simulink model "ModeloBloque"  (R2013a)
settings: Solver=ode45  StartTime=0.0  StopTime=300  RelTol=1e-3
settings Model: Creator=Cristhian Ivan  LastModifiedBy=Cristhian Ivan

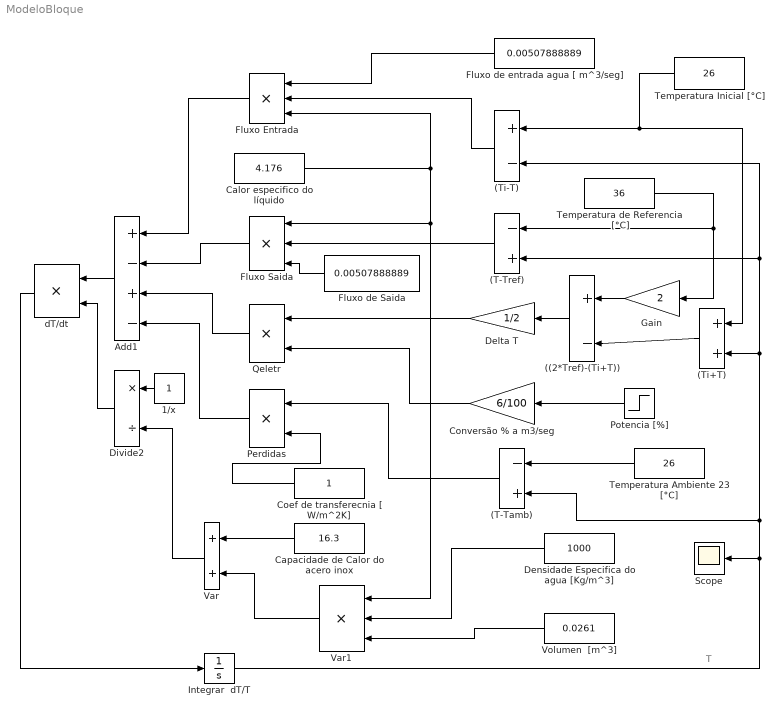
== system ModeloBloque ==
  note: T
  ((2*Tref)-(Ti+T)) : Sum  Inputs=+-
  (T-Tamb) : Sum  Inputs=-+
  (T-Tref) : Sum  Inputs=-+
  (Ti+T) : Sum
  (Ti-T) : Sum  Inputs=+-
  1/x : Constant
  Add1 : Sum  Inputs=+-+-
  Calor especifico do líquido : Constant  Value=4.176
  "Capacidade de Calor do acero inox " : Constant  Value=16.3
  Coef de transferecnia [ W/m^2K] : Constant
  Conversão % a m3/seg : Gain  Gain=6/100
  Delta T : Gain  Gain=1/2
  "Densidade Especifica do agua [Kg/m^3] " : Constant  Value=1000
  Divide2 : Product  Inputs=*/
  Fluxo Entrada : Product  Inputs=***
  Fluxo Saida : Product  Inputs=***
  "Fluxo de Saida  " : Constant  Value=0.00507888889
  Fluxo de entrada agua [ m^3/seg] : Constant  Value=0.00507888889
  Gain : Gain  Gain=2
  Integrar  dT/T : Integrator
  Perdidas : Product  Inputs=**
  Potencia [%] : Step  Time=0  After=30  SampleTime=0
  Qeletr : Product  Inputs=**
  Scope : Scope
      settings: TimeRange=10  YMin=58.165  YMax=58.225
  "Temperatura Ambiente 23 [°C] " : Constant  Value=26
  Temperatura Inicial [°C] : Constant  Value=26
  Temperatura de Referencia  [°C] : Constant  Value=36
  Var : Sum
  Var1 : Product  Inputs=***
  Volumen  [m^3] : Constant  Value=0.0261
  dT/dt : Product  Inputs=**
  wires:
  Add1/1 -> dT/dt/1
  Fluxo Entrada/1 -> Add1/1
  Temperatura Inicial [°C]/1 -> (Ti-T)/1, (Ti+T)/1
  Calor especifico do líquido/1 -> Fluxo Entrada/3, Fluxo Saida/1, Var1/1
  "Densidade Especifica do agua [Kg/m^3] "/1 -> Var1/2
  "Capacidade de Calor do acero inox "/1 -> Var/1
  Var1/1 -> Var/2
  Volumen  [m^3]/1 -> Var1/3
  Potencia [%]/1 -> Conversão % a m3/seg/1
  dT/dt/1 -> Integrar  dT/T/1
  "Fluxo de Saida  "/1 -> Fluxo Saida/3
  Fluxo de entrada agua [ m^3/seg]/1 -> Fluxo Entrada/1
  Perdidas/1 -> Add1/4
  Coef de transferecnia [ W/m^2K]/1 -> Perdidas/2
  "Temperatura Ambiente 23 [°C] "/1 -> (T-Tamb)/1
  (T-Tamb)/1 -> Perdidas/1
  Divide2/1 -> dT/dt/2
  1/x/1 -> Divide2/1
  Var/1 -> Divide2/2
  (Ti-T)/1 -> Fluxo Entrada/2
  (Ti+T)/1 -> ((2*Tref)-(Ti+T))/2
  Gain/1 -> ((2*Tref)-(Ti+T))/1
  ((2*Tref)-(Ti+T))/1 -> Delta T/1
  Qeletr/1 -> Add1/3
  Delta T/1 -> Qeletr/1
  Conversão % a m3/seg/1 -> Qeletr/2
  Temperatura de Referencia  [°C]/1 -> Gain/1, (T-Tref)/1
  Integrar  dT/T/1 -> (T-Tref)/2, (Ti-T)/2, (Ti+T)/2, (T-Tamb)/2, Scope/1
  Fluxo Saida/1 -> Add1/2
  (T-Tref)/1 -> Fluxo Saida/2
